simulink library "Vessel"  (R2023a)
settings: Solver=VariableStepAuto  StartTime=0.0  StopTime=10.0  RelTol=1e-3
undefined symbols (not defined in the file): A_ann_aor, alpha1, alpha2, atrium_ventricle, BSA, control, conversion_factor, DAP, DLVP, DP_close_aor, DP_open_aor, DPP, DRVP, E0, E_max, E_min, E_sa_0, E_sv_0, eta, g, K_vc_aor, K_vo_aor, l, L0, lambda, m1, m2, M_rg_aor, M_st_aor, MAP, MPP, n, P0, p_septum_on_off, p_th_on_off, phi, PVR, Q_max, rho, SAP, SI, sigma, SLVP, SPP, SRVP, SVR, t_delay, Ts, UVV_0, V0, V_0, V_max, V_tot, Y_aorta, Y_control
libraries: $bdroot x100, simulink x39, dspsigops x20, slpidlib x11, eeGeneralControl x2, dspstat3 x1
(part 1 of 4)
settings Model: Creator=emanuele  LastModifiedBy=priya
settings DataIOCC: FinalStateName=final_simstate  InitialState=new_simstate  SaveFinalState=on  SaveOperatingPoint=on
settings OptimizationCC: ReuseModelBlockBuffer=off

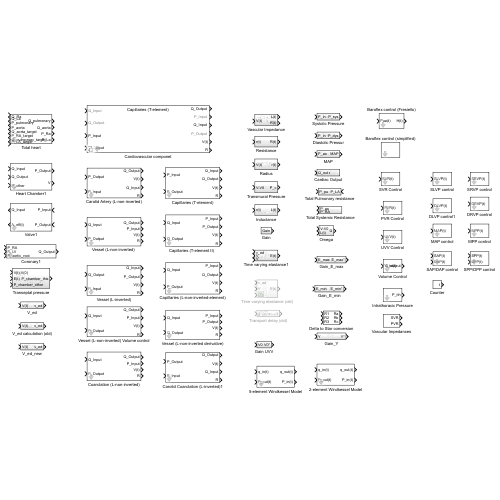
[thumbnail: Simulink's stored preview of the top-level diagram]
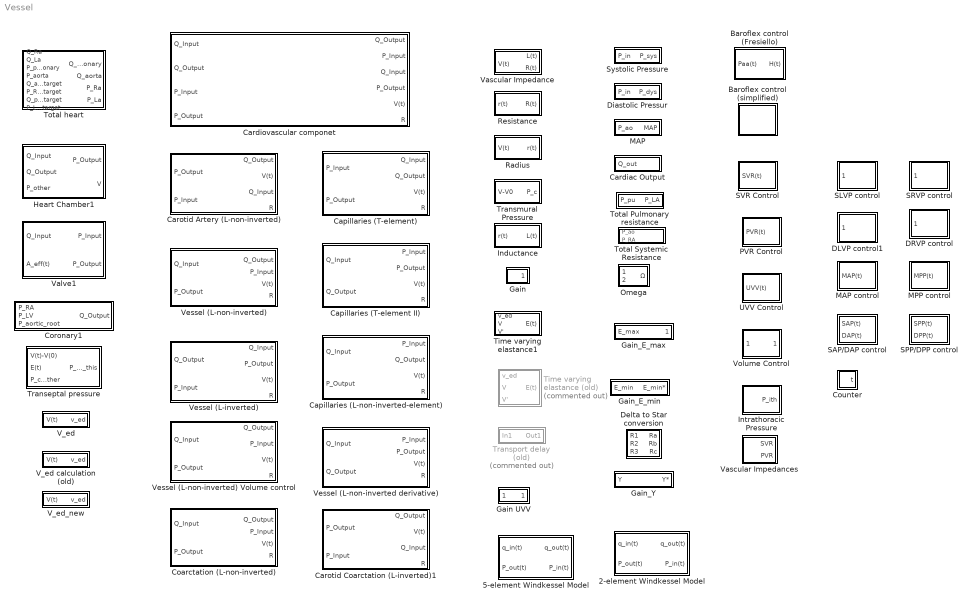
== system Vessel ==
  2-element Windkessel Model : Subsystem  mask{R1=0.001, C1=0.001}
      mask prompts: R1 "R1 (mmHg s/ml)"; C1 "C1 (ml/mmHg)"
      mask DialogControl Descr Prompt: This block models a 2-element windkessel model.
  5-element Windkessel Model : Subsystem  mask{R1=0.001, R2=0.001, C1=0.001, C2=0.001, L=0.001}
      mask prompts: R1 "R1 (mmHg s/ml)"; R2 "R2 (mmHg s/ml)"; C1 "C1 (ml/mmHg)"; C2 "C2 (ml/mmHg)"; L "L (mmHg s^2/ml)"
      mask DialogControl Descr Prompt: This block models a 5-element windkessel model.
  Baroflex control (Fresiello) : Subsystem  mask{C_Hs=-0.09, C_Hv=0.07, D_Hs=2, D_Hv=0.2, T_Hs=2, T_Hv=1.5, H_set=0.7, A=0.242, B=0.12, C=-0.041, D=-0.041, ka=11.758, kes=0.0675, kev=7.06, Fes_0=16.11, Fes_inf=2.10, Fev_0=3.2, Fev_inf0=6.3, Fas_min=2.52, Fas_max=47.78, Paa_SET0=90, tau_p=2.076, tau_z=6.37, WL=0}
      mask prompts: C_Hs "C_Hs: sympathetic control gain for the parameter H (s/(spikes/s))"; C_Hv "C_Hv: vagal control gain for the parameter H (s/(spikes/s))"; D_Hs "D_Hs: sympathetic delay for the parameter H (s)"; D_Hv "D_Hv: vagal delay for the parameter H (s)"; T_Hs "T_Hs: time constant of sympathetic control (s)"; T_Hv "T_Hv: time constant of vagal control (s)"; H_set "H_SET: set point value of H"; A "A: rate pf Paa_SET increase per unit of WL (mmHg/W)"; B "B: rate pf Fes increase per unit of WL (spike/(W⋅s))"; C "C: rate pf Fev decrease per unit of WL (spike/(W·s))"; D "D: rate of Fev_inf decrease per unit of WL (spike/(W·s))"; ka "ka: Fas slope parameter (mmHg)"; kes "kes: Fes slope parameter (s)"; kev "kev: Fev slope parameter (spikes/s)"; Fes_0 "Fes_0: Fes upper limit (spikes/s)"; Fes_inf "Fes_inf: Fes lower limit (spikes/s)"; Fev_0 "Fev_0: Fev lower limit (spikes/s)"; Fev_inf0 "Fev_inf0: Fev upper limit (spikes/s)"; Fas_min "Fas_min: lower saturation of frequency discharge (spikes/s)"; Fas_max "Fas_max: upper saturation of frequency discharge (spikes/s)"; Paa_SET0 "Paa_SET0: set point pressure (mmHg)"; tau_p "tau_p: pole (s)"; tau_z "tau_z: zero (s)"; WL "WL: workload (W)"
      mask init:
      | Fas_0 = Fas_min+Fas_max; %central point of afferent sympathetic activity (spikes/s)
      mask DialogControl DescGroupVar Prompt: Baroflex control with nerve activation function
      mask DialogControl DescTextVar Prompt: The baroreflex model was taken from Ursino (1998) and Fresiello et al. (2013). It provides a representation of the afferent nerve activity, depending on the pressure sensed in the aortic region. In addition, the model reproduces the vagal and sympathetic nerve activity and their effects on cardiovascular parameters. In the model of Ursino (1998) the pressure in the carotid arteries is the input the baroreflex control. Since in the present simulator there is no specific representation of the carotid arteries, the aortic pressure without the effect of the intrathoracic pressure was considered as input pressure for the baroreflex control (Paa).
      mask DialogControl Container5 Prompt: Baroflex parametere for cardiovasculat parameter H(t)
      mask DialogControl Container6 Prompt: General baroflex and nerve parameters
  Baroflex control (simplified) : Subsystem  mask{G_baro=0.003, P_target=110, T_target=0.7, onoff=off}
      mask prompts: G_baro "Baroflex Gain (ms/mmHg)"; P_target "Pressure target (mmHg)"; T_target "Cardiac cycle target (s)"; onoff "Enable"
      mask DialogControl noll Prompt: Baroflex Control Parameters
  Capillaries (L-non-inverted-element) : Subsystem  mask{l=0.02, r=0.0005, h=0.00001, n=11200000000, P0=6}
      mask prompts: l "Length (cm)"; r "Radius (cm)"; h "Thickness (cm)"; n "Number of branches"; P0 "P0 (mmHg)"
      mask init:
      | % rho = 1.060; % g/mL
      | % Y = 3000; % mmHg
      | % eta = 0.00024; % mmHg * s
      | % g = 980.665; % cm / s^2
      | % conversion_factor = 1.3595101283313; %g/cm^2-->mmHg
      | % lambda = 0.5;
      | % V0 = pi*r^2*l*n;
      | % E0 = Y*h/(2*pi*r^3*l*n);
      | % phi = P0/E0;
      | % R0 = eta*8*l/(pi*r^4*n);
      | % L0 = rho * l/ (pi * r^2 * n)/g/conversion_factor;
      mask DialogControl DescGroupVar Prompt: Cardiovascular vessel
      mask DialogControl DescTextVar Prompt: This block models a cardiovascular vessel. Plese choose between L-inverted elelement and not-inverted L-element. Add geomtrical information. Select what variables are input and what are outputs.
      mask DialogControl ParameterGroupVar Prompt: Vessel's Parameters
  "Capillaries (T-element II)  " : Subsystem  mask{l=0.02, r=0.0005, h=0.00001, n=11200000000, P0=6}
      mask prompts: l "Length (cm)"; r "Radius (cm)"; h "Thickness (cm)"; n "Number of branches"; P0 "P0 (mmHg)"
      mask init: same as Vessel/Capillaries (L-non-inverted-element)
      mask DialogControl DescGroupVar Prompt: Cardiovascular vessel
      mask DialogControl DescTextVar Prompt: This block models a cardiovascular vessel. Plese choose between L-inverted elelement and not-inverted L-element. Add geomtrical information. Select what variables are input and what are outputs.
      mask DialogControl ParameterGroupVar Prompt: Vessel's Parameters
  Capillaries (T-element) : Subsystem  mask{l=0.02, r=0.0005, h=0.00001, n=11200000000, P0=6}
      mask prompts: l "Length (cm)"; r "Radius (cm)"; h "Thickness (cm)"; n "Number of branches"; P0 "P0 (mmHg)"
      mask init: same as Vessel/Capillaries (L-non-inverted-element)
      mask DialogControl DescGroupVar Prompt: Cardiovascular vessel
      mask DialogControl DescTextVar Prompt: This block models a cardiovascular vessel. Plese choose between L-inverted elelement and not-inverted L-element. Add geomtrical information. Select what variables are input and what are outputs.
      mask DialogControl ParameterGroupVar Prompt: Vessel's Parameters
  Cardiac Output : Subsystem
  Cardiovascular componet : Subsystem  Variant=on  mask{choice=Capillary compartment (T element), control=None, Y_control=Systemic Arteries, l=2, r=1.6, h=0.163, n=1, P0=80, Y=2000, SI=0, V_tot=V_tot, p_th_on_off=off}
      mask prompts: choice "Windkessel model"; control "Type of control"; Y_control "Young modulus control"; l "Length (cm)"; r "Radius (cm)"; h "Thickness (cm)"; n "Number of branches"; P0 "P0 (mmHg)"; Y "Y (mmHg)"; SI "Stenosis index"; V_tot "V_tot (ml)"; p_th_on_off "Intrathoracic pressure"
      mask init:
      | rho = 1.060; % g/mL
      | %Y =2000; % mmHg
      | eta = 0.00024; % mmHg * s
      | g = 980.665; % cm / s^2
      | conversion_factor = 1.3595101283313; %g/cm^2-->mmHg
      | lambda = 0.5;
      | 
      | %  Scaling to patient's size
      | if V_tot ~=0
      |     k = r/l;                % ratio between radius and length;
      |     V_tot_0 = 4528;
      |     C = V_tot/V_tot_0;
      |     V0 = pi*r^2*l*n;        % Initial volume of original vessel
      |     l = (C*V0/pi/k^2/n)^(1/3);
      |     r = k * l;
      | end
      | 
      | % Calculate volume and impedance
      | V0 = pi*r^2*l*n;
      | E0 = 2*Y*h/(3*pi*r^3*l*n);
      | phi = P0/E0;
      | R0 = eta*8*l/(pi*r^4*n);
      | L0 = rho * l/ (pi * r^2 * n)/g/conversion_factor;
      mask TypeOptions choice: Vessel compartment (L-non-inverted element) | Vessel compartment (L-inverted element) | Capillary compartment (T element) | Capillary compartment (L-non-inverted element) | Capillary compartment (T element II) | Carotid Artery (L-non-inverted) | Vessel (L-non-inverted derivative) | Vessel (volume control)
      mask TypeOptions control: SVR control | PVR control | UVV control | None
      mask TypeOptions Y_control: Systemic Arteries | Systemic Veins | Pulmonary Arteries | Pulmonary Veins | None
      mask DialogControl DescGroupVar Prompt: Cardiovascular vessel
      mask DialogControl DescTextVar Prompt: This block models a cardiovascular vessel. Plese choose between L-inverted elelement and not-inverted L-element. Add geomtrical information. Select what variables are input and what are outputs.
      mask DialogControl ParameterGroupVar Prompt: Vessel's Parameters
  Carotid Artery (L-non-inverted) : Subsystem  mask{l=2, r=1.6, h=0.163, n=1, P0=80}
      mask prompts: l "Length (cm)"; r "Radius (cm)"; h "Thickness (cm)"; n "Number of branches"; P0 "P0 (mmHg)"
      mask init:
      | % rho = 1.060; % g/mL
      | % Y = 2000; % mmHg
      | % eta = 0.00024; % mmHg * s
      | % g = 980.665; % cm / s^2
      | % conversion_factor = 1.3595101283313; %g/cm^2-->mmHg
      | % lambda = 0.5;
      | % V0 = pi*r^2*l*n;
      | % E0 = Y*h/(2*pi*r^3*l*n);
      | % phi = P0/E0;
      | % R0 = eta*8*l/(pi*r^4*n);
      | % L0 = rho * l/ (pi * r^2 * n)/g/conversion_factor;
      mask DialogControl DescGroupVar Prompt: Cardiovascular vessel
      mask DialogControl DescTextVar Prompt: This block models a cardiovascular vessel. Plese choose between L-inverted elelement and not-inverted L-element. Add geomtrical information. Select what variables are input and what are outputs.
      mask DialogControl ParameterGroupVar Prompt: Vessel's Parameters
  Carotid Coarctation (L-inverted)1 : Subsystem  mask{l=2, SI=0, L0=0.5107007067709949, P0=100, Y=2000, Y_control=Systemic arteries}
      mask prompts: l "Length (cm)"; SI "Stenosis index"; L0 "L0 (CGS units)"; P0 "P0 (mmHg)"; Y "Young Modulus (mmhg)"; Y_control "Young modulus control"
      mask init:
      | rho = 1.060; % g/mL
      | control = 4;
      | %Y = 2000; % mmHg
      | eta = 0.00024; % mmHg * s
      | g = 980.665; % cm / s^2
      | conversion_factor = 1.3595101283313; %g/cm^2-->mmHg
      | lambda = 0.5;
      | r = sqrt(rho * l / pi / L0);
      | h = r/10;
      | n = 1;
      | V0 = pi*r^2*l;
      | E0 = Y*h/(2*pi*r^3*l);
      | phi = P0/E0;
      | R0 = eta*8*l/(pi*r^4);
      | L0 = rho * l/ (pi * r^2 )/g/conversion_factor;
      mask TypeOptions Y_control: Systemic arteries | Systemic veins | Pulmonary arteries | Pulmonary veins | None
      mask DialogControl DescGroupVar Prompt: Cardiovascular vessel
      mask DialogControl DescTextVar Prompt: This block models a cardiovascular vessel. Plese choose between L-inverted elelement and not-inverted L-element. Add geomtrical information. Select what variables are input and what are outputs.
      mask DialogControl ParameterGroupVar Prompt: Vessel's Parameters
  Coarctation (L-non-inverted) : Subsystem  mask{l=2, SI=0, L0=0.5107007067709949, P0=100, Y=Y_aorta, Y_control=Systemic Arteries}
      mask prompts: l "Length (cm)"; SI "Stenosis index"; L0 "L0 (CGS units)"; P0 "P0 (mmHg)"; Y "Young Modulus (mmhg)"; Y_control "Young Modulus control"
      mask init:
      | rho = 1.060; % g/mL
      | control = 4;
      | %Y = 2000; % mmHg
      | eta = 0.00024; % mmHg * s
      | g = 980.665; % cm / s^2
      | conversion_factor = 1.3595101283313; %g/cm^2-->mmHg
      | lambda = 0.5;
      | r = sqrt(rho * l / pi / L0);
      | h = r/10;
      | n = 1;
      | V0 = pi*r^2*l;
      | E0 = 2*Y*h/(3*pi*r^3*l);
      | phi = P0/E0;
      | R0 = eta*8*l/(pi*r^4);
      | L0 = rho * l/ (pi * r^2 )/g/conversion_factor;
      mask TypeOptions Y_control: Systemic Arteries | Systemic Veins | Pulmonary Arteries | Pulmonary Veins | None
      mask DialogControl DescGroupVar Prompt: Cardiovascular vessel
      mask DialogControl DescTextVar Prompt: This block models a cardiovascular vessel. Plese choose between L-inverted elelement and not-inverted L-element. Add geomtrical information. Select what variables are input and what are outputs.
      mask DialogControl ParameterGroupVar Prompt: Vessel's Parameters
  Coronary1 : Subsystem  mask{R_ca=0}
  Counter : Subsystem
  DLVP control1 : Subsystem  mask{DLVP_0=DLVP, dt=3, onoff=on}
      mask prompts: DLVP_0 "DLVP tartget"; dt "Time step (s)"; onoff "Enable"
  DRVP control : Subsystem  mask{DRVP_0=DRVP, dt=3, onoff=on}
      mask prompts: DRVP_0 "DRVP tartget"; dt "Time step (s)"; onoff "Enable"
  Delta to Star conversion : Subsystem
  Diastolic Pressur : Subsystem
  Gain : Subsystem
  Gain UVV : Subsystem
  Gain_E_max : Subsystem
  Gain_E_min : Subsystem
  Gain_Y : Subsystem
  Heart Chamber1 : Subsystem  mask{control=Right Atrium, E_max=0.06, E_min=0.04, alpha1=0.1, alpha2=0.2, m1=1.2, m2=10, R_wall=0.0005, t_delay=85e-3, V_0=17, v_o=40, sigma=0.0015, V_max=400, Q_max=2000, T0=0.8, P_pc_0=-2, K_pc=1, V_pc_0=320, V_pe=30, phi_pc=40, E_sa_0=12, E_sv_0=46, atrium_ventricle=Atrium}
      mask prompts: E_max "Maximum elastance (mmHg/mL)"; E_min "Minimum elastance (mmHg/mL)"; alpha1 "α₁"; alpha2 "α₂"; m1 "m₁"; m2 "m₂"; V_0 "Residual volume (mL)"; v_o "Initial volume (mL)"; sigma "σ"; T0 "Cardiac cycle (s)"; P_pc_0 "P_pc₀ (minimal pericardial pressure)"; K_pc "K_pc (pericardial pressure constant"; V_pc_0 "V_pc (pericardial volume constant)"; V_pe "Pericardial fluid volume"; phi_pc "φ_pc (pericardial volume constant)"; E_sa_0 "E_sa₀"; E_sv_0 "E_sv₀"; atrium_ventricle "Chamber"
      mask init:
      | %tau1 = alpha1*T0;
      | %tau2 = alpha2*T0;
      | Q_min = -Q_max;
      | V_min = V_0;
      mask TypeOptions control: Right Atrium | Right Ventricle | Left Atrium | Left Ventricle | None
      mask TypeOptions atrium_ventricle: Atrium | Ventricle
      mask DialogControl ParameterGroupVar Prompt: Heart Chamber Parameters
      mask DialogControl Container4 Prompt: Pericardium Parameters
  Inductance : Subsystem
  Intrathoracic Pressure : Subsystem  mask{t_ins=2, t_exp=3, p_ita=1.8, p_itb=-5.5}
      mask prompts: t_ins "Inspiration cycle (s)"; t_exp "Expiration cycle (s)"; p_ita "Pressure variation (mmHg)"; p_itb "Pressure baseline (mmHg)"
      mask init:
      | tau_insp = t_ins/10;
      | tau_exp = t_exp/10;
      mask DialogControl DescGroupVar Prompt: Intrathoracic pressure
      mask DialogControl DescTextVar Prompt: The parameters for simulating the varying thoracic pressure during the breathing cycle are taken from: A comprehensive model for right-left heart interaction under the influence of pericardium and baroreflex
  MAP : Subsystem
  MAP control : Subsystem  mask{MAP_0=MAP, dt=1, onoff=on}
      mask prompts: MAP_0 "MAP tartget"; dt "Time step (s)"; onoff "Enable"
  MPP control : Subsystem  mask{MPP_0=MPP, dt=3, onoff=on}
      mask prompts: MPP_0 "MPP tartget"; dt "Time step (s)"; onoff "Enable"
  Omega : Subsystem
  PVR Control : Subsystem  mask{PVR_0=PVR, onoff=on}
      mask prompts: PVR_0 "PVR tartget"; onoff "Enable"
  Radius : Subsystem
  Resistance : Subsystem
  SAP/DAP control : Subsystem  mask{SAP_0=SAP, DAP_0=DAP, dt=1, onoff=on}
      mask prompts: SAP_0 "SAP target"; DAP_0 "DAP target"; dt "Time step (s)"; onoff "Enable"
  SLVP control : Subsystem  mask{SLVP_0=SLVP, dt=3, onoff=on}
      mask prompts: SLVP_0 "SLVP tartget"; dt "Time step (s)"; onoff "Enable"
  SPP/DPP control : Subsystem  mask{SPP_0=SPP, DPP_0=DPP, dt=3, onoff=on}
      mask prompts: SPP_0 "SPP target"; DPP_0 "DPP target"; dt "Time step (s)"; onoff "Enable"
  SRVP control : Subsystem  mask{SRVP_0=SRVP, dt=3, onoff=on}
      mask prompts: SRVP_0 "SRVP tartget"; dt "Time step (s)"; onoff "Enable"
  SVR Control : Subsystem  mask{SVR_0=SVR, onoff=on}
      mask prompts: SVR_0 "SVR tartget"; onoff "Enable"
  Systolic Pressure : Subsystem
  Time varying elastance (old) : Subsystem  Commented=on
  Time varying elastance1 : Subsystem
  Total Pulmonary resistance : Subsystem
      settings: PortSchema="{\"entries\":[{\"content\":{\"sides\":[{\"content\":{\"connectorIds\":[\"In1\"]},\"type\":\"ConnectorPlacement.EquallySpacedRectSide\",\"uuid\":\"c9341461-c171-4eac-a287-36e7cd79ba9c\"},{\"content\":{\"connectorIds\":[\"In2\"],\"side\":\"RIGHT\"},\"type\":\"ConnectorPlacement.EquallySpacedRectSide\",\"uuid\":\"dd479575-dfa7-40be-8840-552306c7a812\"},{\"content\":{\"connectorIds\":[],\"side\":\"TOP\"},\"type\":\"ConnectorPlacement.EquallySpacedRectSide\",\"uuid\":\"55fb924b-6719-416a-80e5-0f49fb901268\"}]},\"type\":\"ConnectorPlacement.EquallySpacedConnector\",\"uuid\":\"ed4dd8c3-ddc7-4a34-b37b-80f1af9032bf\"}],\"packageUris\":[\"http://schema.mathworks.com/mf0/Connector/R2020b\"],\"version\":\"1.0\"}"
  Total Systemic Resistance : Subsystem
  Total heart : Subsystem  mask{BSA=BSA, T0=0.833, R_lca=40, R_rca=80, p_septum_on_off=on, E_max_ra=0.15, E_max_rv=0.6, E_max_la=0.17, E_max_lv=3, E_min_ra=0.04, E_min_rv=0.04, E_min_la=0.08, E_min_lv=0.09, alpha1_ra=0.1, alpha1_rv=0.2, alpha1_la=0.1, alpha1_lv=0.2, alpha2_ra=0.2, alpha2_rv=0.25, alpha2_la=0.2, alpha2_lv=0.25, m1_ra=1.2, m1_rv=1.2, m1_la=1.2, m1_lv=1.2, m2_ra=10, m2_rv=10, m2_la=10, m2_lv=20, R_wall_ra=0.0005, R_wall_rv=0.00020, R_wall_la=0.00050, R_wall_lv=0.00005, t_delay_ra=85e-3, t_delay_rv=245e-3, t_delay_la=95e-3, t_delay_lv=245e-3, V_0_ra=17, V_0_rv=55, V_0_la=3, V_0_lv=5, v_o_ra=60, v_o_rv=100, v_o_la=60, v_o_lv=40, sigma_ra=0.0015, sigma_rv=0.0030, sigma_la=0.0015, sigma_lv=0.003, V_max_ra=400, V_max_rv=400, V_max_la=400, V_max_lv=400, Q_max_ra=4000, Q_max_rv=2000, Q_max_la=4000, Q_max_lv=2000, A_ann_tri=7.7, A_ann_pul=1.5^2*pi, A_ann_mit=7.7, A_ann_aor=1.6^2*pi, K_vo_tri=40, K_vo_pul=30, K_vo_mit=40, K_vo_aor=20, K_vc_tri=30, K_vc_pul=30, K_vc_mit=20, K_vc_aor=20, M_st_tri=1, M_st_pul=1, M_st_mit=1, M_st_aor=1, M_rg_tri=0, M_rg_pul=0, M_rg_mit=0, M_rg_aor=0, DP_open_tri=0, DP_open_pul=0, DP_open_mit=0, DP_open_aor=0, DP_close_tri=0, DP_close_pul=0, DP_close_mit=0, DP_close_aor=0, P_pc_0=-2, K_pc=1, V_pc_0=320, V_pe=30, phi_pc=50, E_sa_0=12, E_sv_0=46}
      mask prompts: BSA "BSA (m^2)"; T0 "Cardiac cycle (s)"; R_lca "Left coronary artery resistance"; R_rca "Right coronary artery resistance"; p_septum_on_off "Atrial/Ventricular septum"; P_pc_0 "P_pc₀ (minimal pericardial pressure)"; K_pc "K_pc (pericardial pressure constant"; V_pc_0 "V_pc (pericardial volume constant)"; V_pe "Pericardial fluid volume"; phi_pc "φ_pc (pericardial volume constant)"; E_sa_0 "E_sa₀"; E_sv_0 "E_sv₀"
      mask init:
      | %General
      | if BSA~=0
      |     
      | V_0_ra      =   BSA^(1.0974) * 5.1668;
      | V_0_rv      =   BSA^(1.0974) * 5.1668;
      | 
      | sigma_ra    =   BSA^(-1.0849) * 0.0029;
      | sigma_la    =   BSA^(-1.0849) * 0.0029;
      | sigma_rv    =   BSA^(-1.0522) * 0.0188;
      | sigma_lv    =   BSA^(-1.0522) * 0.0188;
      | 
      | V_max_ra    =   BSA^(1.0971) * 129.3569;
      | V_max_la    =   BSA^(1.0971) * 129.3569;
      | V_max_rv    =   BSA^(1.0956) * 181.1664;
      | V_max_lv    =   BSA^(1.0956) * 181.1664;
      | 
      | Q_max_ra    =   BSA^(1.0955) * 2070.9;
      | Q_max_la    =   BSA^(1.0955) * 2070.9;
      | Q_max_rv    =   BSA^(1.0965) * 1034.8;
      | Q_max_lv    =   BSA^(1.0965) * 1034.8;
      | 
      | V_pe        =   BSA^(1.1720) * 14.7750;
      | V_pc_0      =   BSA^(1.3765) * 127.1945;
      | phi_pc      =   BSA^(1.1152) * 25.6292;
      | E_sa_0      =   BSA^(-1.0014) * 18.5433;
      | E_sv_0      =   BSA^(-1.0014) * 18.5433;
      | 
      | end
      mask DialogControl Container7 Prompt: General Parameters
      mask DialogControl Container9 Prompt: General Parameters
      mask DialogControl Container8 Prompt: Chambers parameters
      mask DialogControl Container15 Prompt: Chambers parameters
      mask DialogControl Control1_copy_copy_copy_copy_copy_copy Prompt: Parameter
      mask DialogControl Control1_copy_copy_copy Prompt: Right atrium
      mask DialogControl Control1_copy_copy_copy_copy Prompt: Right ventricle
      mask DialogControl Control1_copy_copy_copy_copy_copy Prompt: Left Atrium
      mask DialogControl Control1_copy Prompt: Left Ventricle
      mask DialogControl Control6 Prompt: E_max
      mask DialogControl Control7 Prompt: E_min
      mask DialogControl Control8 Prompt: α₁
      mask DialogControl Control9 Prompt: α₂
      mask DialogControl Control10 Prompt: m₁
      mask DialogControl Control11 Prompt: m₂
      mask DialogControl Control12 Prompt: R_wall
      mask DialogControl Control13 Prompt: t_delay
      mask DialogControl Control14 Prompt: V₀
      mask DialogControl Control15 Prompt: v₀
      mask DialogControl Control16 Prompt: σ
      mask DialogControl Control15_copy Prompt: V_max
      mask DialogControl Control15_copy_copy Prompt: Q_max
      mask DialogControl Container10 Prompt: Valves Parameters
      mask DialogControl Container5 Prompt: Valves Parameters
      mask DialogControl Control17 Prompt: Parameter
      mask DialogControl Control18 Prompt: Tricuspid valve
      mask DialogControl Control18_copy Prompt: Pulmonary valve
      mask DialogControl Control18_copy_copy Prompt: Mitral valve
      mask DialogControl Control18_copy_copy_copy Prompt: Aortic valve
      mask DialogControl Control22 Prompt: A_ann
      mask DialogControl Control23 Prompt: K_vo
      mask DialogControl Control24 Prompt: K_vc
      mask DialogControl Control25 Prompt: M_st
      mask DialogControl Control26 Prompt: M_rg
      mask DialogControl Control27 Prompt: Δp_open
      mask DialogControl Control28 Prompt: Δp_close
      mask DialogControl Container11 Prompt: Pericardium Parameters
      mask DialogControl Container4 Prompt: Pericardium Parameters
  Transeptal pressure : Subsystem
  Transmural Pressure : Subsystem
  Transport delay (old) : Subsystem  Commented=on
  UVV Control : Subsystem  mask{UVV_0=3400, onoff=on}
      mask prompts: UVV_0 "UVV tartget"; onoff "Enable"
  V_ed : Subsystem
  V_ed calculation (old) : Subsystem
  V_ed_new : Subsystem
  Valve1 : Subsystem  mask{A_ann=A_ann_aor, K_vo=K_vo_aor, K_vc=K_vc_aor, M_st=M_st_aor, M_rg=M_rg_aor, DP_open=DP_open_aor, DP_close=DP_close_aor, Q_max=4000, Q_min=0}
      mask prompts: A_ann "Area (cm^2)"; K_vo "Opening constant (1/mmHg/s)"; K_vc "Closing constant (1/mmHg/s)"; M_st "Stenosis index"; M_rg "Regurgitation index"; DP_open "Opening pressure gradient (mmHg)"; DP_close "Closing pressure gradient (mmHg)"; Q_max "Maximum flow"; Q_min "Minimum flow"
      mask init:
      | rho = 1.060; %g/cm^3
  Vascular Impedance : Subsystem
  Vascular Impedances : Subsystem
  Vessel (L-inverted) : Subsystem  mask{l=2, r=1.6, h=0.163, n=1, P0=80}
      mask prompts: l "Length (cm)"; r "Radius (cm)"; h "Thickness (cm)"; n "Number of branches"; P0 "P0 (mmHg)"
      mask init: same as Vessel/Capillaries (L-non-inverted-element)
      mask DialogControl DescGroupVar Prompt: Cardiovascular vessel
      mask DialogControl DescTextVar Prompt: This block models a cardiovascular vessel. Plese choose between L-inverted elelement and not-inverted L-element. Add geomtrical information. Select what variables are input and what are outputs.
      mask DialogControl ParameterGroupVar Prompt: Vessel's Parameters
  Vessel (L-non-inverted derivative) : Subsystem  mask{l=2, r=1.6, h=0.163, n=1, P0=80}
      mask prompts: l "Length (cm)"; r "Radius (cm)"; h "Thickness (cm)"; n "Number of branches"; P0 "P0 (mmHg)"
      mask init:
      | % rho = 1.060; % g/mL
      | % Y = 3000; % mmHg
      | % eta = 0.00024; % mmHg * s
      | % g = 980.665; % cm / s^2
      | % conversion_factor = 1.3595101283313; %g/cm^2-->mmHg
      | % lambda = 0.5;
      | % V0 = pi*r^2*l*n;
      | % E0 = Y*h/(2*pi*r^3*l*n);
      | % phi = P0/E0;
      | % R0 = eta*8*l/(pi*r^4*n);
      | % L0 = rho * l/ (pi * r^2 * n)/g/conversion_factor;
      mask DialogControl DescGroupVar Prompt: Cardiovascular vessel
      mask DialogControl DescTextVar Prompt: This block models a cardiovascular vessel. Plese choose between L-inverted elelement and not-inverted L-element. Add geomtrical information. Select what variables are input and what are outputs.
      mask DialogControl ParameterGroupVar Prompt: Vessel's Parameters
  "Vessel (L-non-inverted) " : Subsystem  mask{l=2, r=1.6, h=0.163, n=1, P0=80}
      mask prompts: l "Length (cm)"; r "Radius (cm)"; h "Thickness (cm)"; n "Number of branches"; P0 "P0 (mmHg)"
      mask init: same as Vessel/Vessel (L-non-inverted derivative)
      mask DialogControl DescGroupVar Prompt: Cardiovascular vessel
      mask DialogControl DescTextVar Prompt: This block models a cardiovascular vessel. Plese choose between L-inverted elelement and not-inverted L-element. Add geomtrical information. Select what variables are input and what are outputs.
      mask DialogControl ParameterGroupVar Prompt: Vessel's Parameters
  Vessel (L-non-inverted) Volume control : Subsystem  mask{l=2, r=1.6, h=0.163, n=1, P0=80}
      mask prompts: l "Length (cm)"; r "Radius (cm)"; h "Thickness (cm)"; n "Number of branches"; P0 "P0 (mmHg)"
      mask init: same as Vessel/Vessel (L-non-inverted derivative)
      mask DialogControl DescGroupVar Prompt: Cardiovascular vessel
      mask DialogControl DescTextVar Prompt: This block models a cardiovascular vessel. Plese choose between L-inverted elelement and not-inverted L-element. Add geomtrical information. Select what variables are input and what are outputs.
      mask DialogControl ParameterGroupVar Prompt: Vessel's Parameters
  Volume Control : Subsystem  mask{V_tot_0=4800}
      mask prompts: V_tot_0 "Total blood volume (mL)"

== system Vessel/2-element Windkessel Model ==
  note: 2-element Windkessel Model
  q_in(t) : Inport
  P_out(t) : Inport  Port=2
  Bias : Bias  Bias=0.0  SaturateOnIntegerOverflow=off
  Gain3 : Gain  Gain=1/C1
  Gain4 : Gain  Gain=1/R1
  Minus3 : Sum  Inputs=+-
  Minus4 : Sum  Inputs=-+
  P_1(t) : Integrator
  q_out(t) : Outport
  P_in(t) : Outport  Port=2
  wires:
  Minus4/1 -> Gain4/1
  P_out(t)/1 -> Minus4/1  "P_out(t)"
  P_1(t)/1 -> Bias/1  "P_1(t)"
  Gain3/1 -> P_1(t)/1  "P_1(t)'"
  Minus3/1 -> Gain3/1  "q_1(t)"
  Gain4/1 -> Minus3/2, q_out(t)/1  "q_out(t)"
  q_in(t)/1 -> Minus3/1  "q_in(t)"
  Bias/1 -> P_in(t)/1, Minus4/2

== system Vessel/5-element Windkessel Model ==
  note: 5-element Windkessel Model
  q_in(t) : Inport
  P_out(t) : Inport  Port=2
  Bias : Bias  Bias=0.0  SaturateOnIntegerOverflow=off
  Bias1 : Bias  Bias=0.0  SaturateOnIntegerOverflow=off
  Gain : Gain  Gain=R1
  Gain1 : Gain  Gain=1/C1
  Gain2 : Gain  Gain=1/L
  Gain3 : Gain  Gain=1/C2
  Gain4 : Gain  Gain=1/R2
  Minus : Sum  Inputs=-+
  Minus1 : Sum
  Minus2 : Sum  Inputs=+-
  Minus3 : Sum  Inputs=+-
  Minus4 : Sum  Inputs=-+
  P_2(t) : Integrator
  P_C1(t) : Integrator
  Unit Delay : UnitDelay  SampleTime=-1  HasFrameUpgradeWarning=on
  q_L(t) : Integrator
  q_out(t) : Outport
  P_in(t) : Outport  Port=2
  wires:
  Minus/1 -> Gain1/1, Gain/1  "q_1(t)"
  q_in(t)/1 -> Minus/2  "q_in(t)"
  P_C1(t)/1 -> Bias1/1  "P_C1(t)"
  Gain/1 -> Unit Delay/1  "P_R1(t)"
  Gain1/1 -> P_C1(t)/1  "P_C1(t)'"
  Minus1/1 -> P_in(t)/1, Minus2/1  "P_1(t)"
  Minus2/1 -> Gain2/1  "P_1(t)"
  Gain2/1 -> q_L(t)/1  "q_L(t)'"
  q_L(t)/1 -> Minus3/1, Minus/1  "q_L(t)"
  Gain4/1 -> q_out(t)/1, Minus3/2  "q_out(t)"
  Minus3/1 -> Gain3/1  "q_2(t)"
  Gain3/1 -> P_2(t)/1  "P_2(t)'"
  P_2(t)/1 -> Bias/1  "P_2(t)"
  P_out(t)/1 -> Minus4/1  "P_out(t)"
  Minus4/1 -> Gain4/1  "q_out(t)"
  Unit Delay/1 -> Minus1/2
  Bias/1 -> Minus4/2, Minus2/2
  Bias1/1 -> Minus1/1

== system Vessel/Baroflex control (Fresiello) ==
  Paa(t) : Inport
  Afferent sympathetic activity : Subsystem
  Constant : Constant  Value=H_set
  Efferent sympathetic nerve activity : Subsystem
  Efferent vagal nerve activity : Subsystem
  Gain : Gain  Gain=1/T_Hs
  Gain1 : Gain  Gain=1/T_Hv
  Integrator : Integrator
  Integrator1 : Integrator
  Minus : Sum  Inputs=-+|
  Minus1 : Sum  Inputs=+++
  Minus2 : Sum  Inputs=|+-
  Pressure derivation : Subsystem
  Static sympathetic function : Subsystem
  Static vagal function : Subsystem
  XY Graph : Record  FileSettingsInternal="{\"entries\":[{\"content\":{\"excelSettings\":{\"content\":{},\"type\":\"Streamout.ExcelSettings\"}},\"type\":\"Streamout.FileSettingStorage\",\"uuid\":\"\"}],\"packageUris\":[\"http:\\/\\/schema.mathworks.com\\/mf0\\/streamout_blocks\\/R2020a\"],\"version\":\"1.0\"}"  Layout=[1 1]  SignalsInternal="{\"entries\":[{\"content\":{\"signals\":[{\"content\":{\"blockPath\":[],\"dimensions\":[1],\"domain\":\"\",\"lineColor\":\"#a2142f\",\"plots\":[1],\"port\":1,\"signalID\":8,\"signalName\":\"XY Graph:1\"},\"type\":\"RecordBlkView.Signal\",\"uuid\":\"\"},{\"content\":{\"blockPath\":[],\"dimensions\":[1],\"domain\":\"\",\"lineColor\":\"#139fff\",\"plots\":[1],\"port\":2,\"signalID\":11,\"signalName\":\"XY Graph:2\"},\"type\":\"RecordBlkView.Signal\",\"uuid\":\"\"}]},\"type\":\"RecordBlkView.InputSignals\",\"uuid\":\"\"}],\"packageUris\":[\"http:\\/\\/schema.mathworks.com\\/mf0\\/streamout_blocks\\/R2020a\"],\"version\":\"1.0\"}"  VisualizationBindings="{\"xyplotplugin\":{\"info\":[{\"series\":[{\"bindingParametersList\":[{\"parameter\":\"X-Axis\",\"signalID\":8,\"signalName\":\"XY Graph:1\"},{\"parameter\":\"Y-Axis\",\"signalID\":11,\"signalName\":\"XY Graph:2\"}],\"seriesID\":30739}],\"subplotID\":1}]}}"  CompatibilityTag=XY
  H(t) : Outport
  wires:
  Minus1/1 -> H(t)/1
  Constant/1 -> Minus1/2
  Minus/1 -> Gain/1
  Integrator/1 -> Minus/1, Minus1/1  "ΔH_s(t)"
  Static sympathetic function/1(sf_Hs(t)) -> Minus/2  "sf_Hs(t)"
  Gain/1 -> Integrator/1  "ΔH_s(t)'"
  Gain1/1 -> Integrator1/1  "ΔH_v(t)'"
  Static vagal function/1(sf_Hv(t)) -> Minus2/1  "sf_Hv(t)"
  Integrator1/1 -> Minus1/3, Minus2/2  "ΔH_v(t)"
  Minus2/1 -> Gain1/1
  Efferent sympathetic nerve activity/1(" Fes(t)") -> Static sympathetic function/1(Fes(t))  "Fes(t)"
  Efferent vagal nerve activity/1(" Fev(t)") -> Static vagal function/1(Fev(t))  "Fev(t)"
  Afferent sympathetic activity/1(Fas(t)) -> XY Graph/1, Efferent sympathetic nerve activity/1(Fas(t)), Efferent vagal nerve activity/1(Fas(t))
  Pressure derivation/1(P(t)) -> XY Graph/2, Afferent sympathetic activity/1(P(t))
  Paa(t)/1 -> Pressure derivation/1(Paa(t))

== system Vessel/Baroflex control (simplified) ==
  Constant : Constant  Value=P_target
  Constant1 : Constant  Value=T_target
  Constant2 : Constant  Value=onoff
  Data Store Read : DataStoreRead  DataStoreName=T  IndexOptions=Index vector (dialog)  Indices=1  OutputSizes=1
  Data Store Write : DataStoreWrite  DataStoreName=T  IndexOptions=Index vector (dialog)  Indices=1  OutputSizes=1
  Gain : Gain  Gain=G_baro
  Minus : Sum  Inputs=+-
  Minus1 : Sum
  Switch : Switch  Criteria=u2 > Threshold  SaturateOnIntegerOverflow=off  InputSameDT=off
  wires:
  Minus1/1 -> Switch/1
  [P_sys] -> Minus/1
  Constant/1 -> Minus/2
  Gain/1 -> Minus1/1
  Constant1/1 -> Minus1/2
  Minus/1 -> Gain/1
  Constant2/1 -> Switch/2
  Data Store Read/1 -> Switch/3
  Switch/1 -> Data Store Write/1

== system Vessel/Capillaries (L-non-inverted-element) ==
  Q_Input : Inport
  P_Output : Inport  Port=2  Unit=mmHg
  "   " : Sum  Inputs=-+
  Add : Sum  Inputs=+-
  Add1 : Sum  Inputs=+++
  Constant1 : Constant  Value=V0
  Delay : Delay  DelayLength=1
  Divide : Product  Inputs=*/
  Gain UVV : $bdroot/Gain UVV  SystemSampleTime=-1  VariantActivationTime=update diagram  Latency=0  AutoFrameSizeCalculation=off
  Gain1 : Gain  Gain=p_th_on_off
  IC : InitialCondition  Value=0
  IC1 : InitialCondition  Value=P0
  IC2 : InitialCondition  Value=0
  Integrator : Integrator  InitialConditionSource=external  LimitOutput=on  LowerSaturationLimit=0  ContinuousStateAttributes='Volume'
  Omega : $bdroot/Omega  SystemSampleTime=-1  VariantActivationTime=update diagram  Latency=0  AutoFrameSizeCalculation=off
  Product4 : Product
  Saturation : Saturate  UpperLimit=4000  LowerLimit=-4000
  Subtract : Sum  Inputs=+-
  Transmural Pressure : $bdroot/Transmural Pressure  SystemSampleTime=-1  VariantActivationTime=update diagram  Latency=0  AutoFrameSizeCalculation=off
  Vascular Impedance : $bdroot/Vascular Impedance  SystemSampleTime=-1  VariantActivationTime=update diagram  Latency=0  AutoFrameSizeCalculation=off
  P_Input : Outport
  Q_Output : Outport  Port=2
  V(t) : Outport  Port=3
  R : Outport  Port=4
  wires:
  "   "/1 -> Integrator/1, IC2/1  "V(t)'"
  Integrator/1 -> V(t)/1, Add/1  "V(t)"
  Add/1 -> Transmural Pressure/1  "V-V0"
  Transmural Pressure/1 -> Add1/1  "P_c"
  Product4/1 -> Add1/2  "P_Ω"
  Omega/1 -> Product4/1  "Ω"
  Add1/1 -> IC1/1, Subtract/1
  P_Output/1 -> Subtract/2
  Subtract/1 -> Divide/1
  Constant1/1 -> Gain UVV/1
  Divide/1 -> Saturation/1, Delay/1
  [P_ith] -> Gain1/1
  Gain1/1 -> Add1/3
  IC1/1 -> P_Input/1
  IC/1 -> "   "/1
  IC2/1 -> Product4/2
  Delay/1 -> IC/1
  Saturation/1 -> Q_Output/1
  Q_Input/1 -> "   "/2
  Vascular Impedance/2 -> R/1, Divide/2
  Gain UVV/1 -> Integrator/2, Vascular Impedance/1, Add/2

== system Vessel/Capillaries (T-element II)   ==
  "Q_Input " : Inport  Unit=mL/s
  "Q_Output " : Inport  Port=2  Unit=mL/s
  "   " : Sum  Inputs=+-
  Add : Sum  Inputs=+-
  Add1 : Sum
  Add2 : Sum  Inputs=+-
  Add3 : Sum
  Constant1 : Constant  Value=V0
  Delay : Delay  DelayLength=1
  Gain UVV : $bdroot/Gain UVV  SystemSampleTime=-1  VariantActivationTime=update diagram  Latency=0  AutoFrameSizeCalculation=off
  Gain2 : Gain  Gain=1/2
  IC : InitialCondition  Value=0
  Integrator : Integrator  InitialConditionSource=external  LimitOutput=on  LowerSaturationLimit=0  ContinuousStateAttributes='Volume'
  Omega : $bdroot/Omega  SystemSampleTime=-1  VariantActivationTime=update diagram  Latency=0  AutoFrameSizeCalculation=off
  Product : Product
  Product1 : Product
  Product4 : Product
  Transmural Pressure : $bdroot/Transmural Pressure  SystemSampleTime=-1  VariantActivationTime=update diagram  Latency=0  AutoFrameSizeCalculation=off
  Vascular Impedance : $bdroot/Vascular Impedance  SystemSampleTime=-1  VariantActivationTime=update diagram  Latency=0  AutoFrameSizeCalculation=off
  P_Input : Outport
  P_Output : Outport  Port=2  Unit=mmHg
  V(t) : Outport  Port=3
  R : Outport  Port=4
  wires:
  Add2/1 -> P_Output/1
  Add3/1 -> P_Input/1
  "Q_Output "/1 -> Product/1, "   "/2
  "Q_Input "/1 -> "   "/1, Product1/1
  "   "/1 -> Integrator/1, IC/1  "V(t)'"
  Integrator/1 -> Add/1, V(t)/1  "V(t)"
  Add/1 -> Transmural Pressure/1  "V-V0"
  Add1/1 -> Add3/2, Add2/1
  Transmural Pressure/1 -> Add1/1  "P_c"
  Product4/1 -> Add1/2  "P_Ω"
  Omega/1 -> Product4/1  "Ω"
  Constant1/1 -> Gain UVV/1
  Product1/1 -> Add3/1
  Product/1 -> Add2/2
  Delay/1 -> Product4/2
  IC/1 -> Delay/1
  Gain2/1 -> Product1/2, Product/2
  Vascular Impedance/2 -> R/1, Gain2/1
  Gain UVV/1 -> Vascular Impedance/1, Add/2, Integrator/2

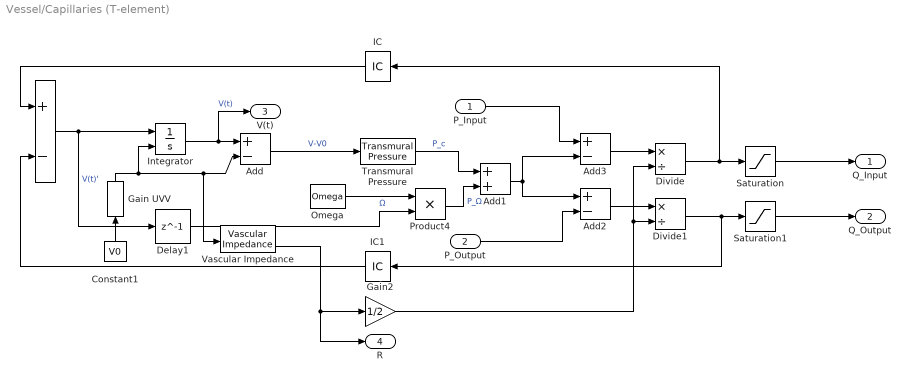
== system Vessel/Capillaries (T-element) ==
  P_Input : Inport
  P_Output : Inport  Port=2
  "   " : Sum  Inputs=+-
  Add : Sum  Inputs=+-
  Add1 : Sum
  Add2 : Sum  Inputs=+-
  Add3 : Sum  Inputs=+-
  Constant1 : Constant  Value=V0
  Delay1 : Delay  DelayLength=1
  Divide : Product  Inputs=*/
  Divide1 : Product  Inputs=*/
  Gain UVV : $bdroot/Gain UVV  SystemSampleTime=-1  VariantActivationTime=update diagram  Latency=0  AutoFrameSizeCalculation=off
  Gain2 : Gain  Gain=1/2
  IC : InitialCondition  Value=0
  IC1 : InitialCondition  Value=0
  Integrator : Integrator  InitialConditionSource=external  LimitOutput=on  LowerSaturationLimit=0  ContinuousStateAttributes='Volume'
  Omega : $bdroot/Omega  SystemSampleTime=-1  VariantActivationTime=update diagram  Latency=0  AutoFrameSizeCalculation=off
  Product4 : Product
  Saturation : Saturate  UpperLimit=4000  LowerLimit=-4000
  Saturation1 : Saturate  UpperLimit=4000  LowerLimit=-4000
  Transmural Pressure : $bdroot/Transmural Pressure  SystemSampleTime=-1  VariantActivationTime=update diagram  Latency=0  AutoFrameSizeCalculation=off
  Vascular Impedance : $bdroot/Vascular Impedance  SystemSampleTime=-1  VariantActivationTime=update diagram  Latency=0  AutoFrameSizeCalculation=off
  Q_Input : Outport
  Q_Output : Outport  Port=2  Unit=mmHg
  V(t) : Outport  Port=3
  R : Outport  Port=4
  wires:
  Constant1/1 -> Gain UVV/1
  Omega/1 -> Product4/1  "Ω"
  Product4/1 -> Add1/2  "P_Ω"
  Transmural Pressure/1 -> Add1/1  "P_c"
  Add1/1 -> Add2/1, Add3/2
  Add/1 -> Transmural Pressure/1  "V-V0"
  Integrator/1 -> V(t)/1, Add/1  "V(t)"
  "   "/1 -> Delay1/1, Integrator/1  "V(t)'"
  Add3/1 -> Divide/1
  Add2/1 -> Divide1/1
  IC/1 -> "   "/1
  IC1/1 -> "   "/2
  P_Input/1 -> Add3/1
  P_Output/1 -> Add2/2
  Delay1/1 -> Product4/2
  Gain2/1 -> Divide1/2, Divide/2
  Divide/1 -> Saturation/1, IC/1
  Divide1/1 -> Saturation1/1, IC1/1
  Saturation1/1 -> Q_Output/1
  Saturation/1 -> Q_Input/1
  Vascular Impedance/2 -> R/1, Gain2/1
  Gain UVV/1 -> Vascular Impedance/1, Add/2, Integrator/2

== system Vessel/Cardiac Output ==
  Q_out : Inport
  Data Store Read1 : DataStoreRead  DataStoreName=T  IndexOptions=Index vector (dialog)  Indices=1  OutputSizes=1
  Divide : Product  Inputs=/*
  Gain2 : Gain  Gain=60
  Integrator1 : Integrator  ExternalReset=falling
  Pulse Generator : DiscretePulseGenerator  PulseType=Time based  TimeSource=Use external signal  Period=100  PulseWidth=1e-3
  Sample and Hold : dspsigops/Sample and Hold  trig=Rising edge  initCond=0  latchinput=off
  To Workspace1 : ToWorkspace  VariableName=SV  SampleTime=-1
  To Workspace4 : ToWorkspace  VariableName=CO  SampleTime=-1
  tag scope: CO=global, Stroke_volume=global
  wires:
  Divide/1 -> [CO], To Workspace4/1
  Data Store Read1/1 -> Divide/1
  Gain2/1 -> Divide/2
  Q_out/1 -> Integrator1/1
  Pulse Generator/1 -> Sample and Hold/Trigger, Integrator1/2
  [t_b] -> Pulse Generator/1
  Integrator1/1 -> Sample and Hold/1
  Sample and Hold/1 -> [Stroke_volume], To Workspace1/1, Gain2/1

== system Vessel/Cardiovascular componet ==
  note: 1) Add Subsystem or Model blocks as valid variant choices.
      | 2) You cannot connect blocks at this level. At simulation, connectivity is automatically
      | determined, based on the active variant and port name matching.
  Q_Input : Inport
  Q_Output : Inport  Port=2
  P_Input : Inport  Port=3
  P_Output : Inport  Port=4
  Capillaries (L-non-inverted-element) : $bdroot/Capillaries (L-non-inverted-element)  VariantControl=choice == 4  l=l  r=r  h=h  n=n  P0=P0
  "Capillaries (T-element II)  " : $bdroot/Capillaries (T-element II)    VariantControl=choice == 5  l=l  r=r  h=h  n=n  P0=P0
  Capillaries (T-element) : $bdroot/Capillaries (T-element)  VariantControl=choice == 3  l=l  r=r  h=h  n=n  P0=P0
  Carotid Artery (L-non-inverted) : $bdroot/Carotid Artery (L-non-inverted)  VariantControl=choice == 6  l=l  r=r  h=h  n=n  P0=P0
  Vessel (L-inverted) : $bdroot/Vessel (L-inverted)  VariantControl=choice == 2  l=l  r=r  h=h  n=n  P0=P0
  Vessel (L-non-inverted derivative) : $bdroot/Vessel (L-non-inverted derivative)  VariantControl=choice == 7  l=l  r=r  h=h  n=n  P0=P0
  "Vessel (L-non-inverted) " : $bdroot/Vessel (L-non-inverted)   VariantControl=choice == 1  l=l  r=r  h=h  n=n  P0=P0
  Vessel (L-non-inverted) Volume control : $bdroot/Vessel (L-non-inverted) Volume control  VariantControl=choice == 8  l=l  r=r  h=h  n=n  P0=P0
  "Q_Output " : Outport
  "P_Input " : Outport  Port=2
  "Q_Input " : Outport  Port=3
  "P_Output " : Outport  Port=4
  V(t) : Outport  Port=5
  R : Outport  Port=6

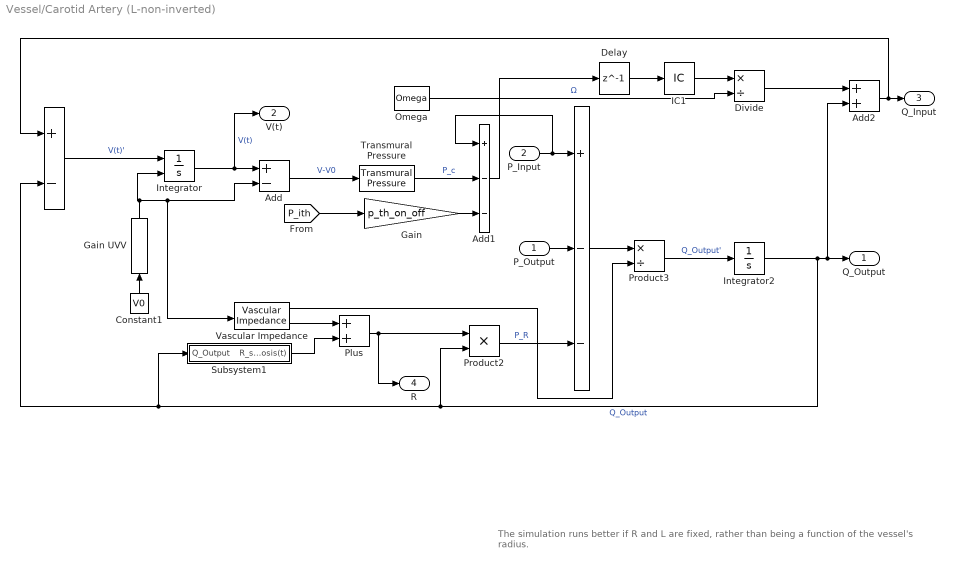
== system Vessel/Carotid Artery (L-non-inverted) ==
  note: The simulation runs better if R and L are fixed, rather than being a function of the vessel's radius.
  P_Output : Inport  Unit=mmHg
  P_Input : Inport  Port=2
  " " : Sum  Inputs=+--
  "   " : Sum  Inputs=+-
  Add : Sum  Inputs=+-
  Add1 : Sum  Inputs=+--
  Add2 : Sum
  Constant1 : Constant  Value=V0
  Delay : Delay  DelayLength=1  InitialCondition=P0
  Divide : Product  Inputs=*/
  Gain : Gain  Gain=p_th_on_off
  Gain UVV : $bdroot/Gain UVV  SystemSampleTime=-1  VariantActivationTime=update diagram  Latency=0  AutoFrameSizeCalculation=off
  IC1 : InitialCondition  Value=P0
  Integrator : Integrator  InitialConditionSource=external  LimitOutput=on  LowerSaturationLimit=0  ContinuousStateAttributes='Volume'
  Integrator2 : Integrator  LimitOutput=on  UpperSaturationLimit=4000  LowerSaturationLimit=-4000  ContinuousStateAttributes='Flow'
  Omega : $bdroot/Omega  SystemSampleTime=-1  VariantActivationTime=update diagram  Latency=0  AutoFrameSizeCalculation=off
  Plus : Sum
  Product2 : Product
  Product3 : Product  Inputs=*/
  Subsystem1 : Subsystem
  Transmural Pressure : $bdroot/Transmural Pressure  SystemSampleTime=-1  VariantActivationTime=update diagram  Latency=0  AutoFrameSizeCalculation=off
  Vascular Impedance : $bdroot/Vascular Impedance  SystemSampleTime=-1  VariantActivationTime=update diagram  Latency=0  AutoFrameSizeCalculation=off
  Q_Output : Outport
  V(t) : Outport  Port=2
  Q_Input : Outport  Port=3
  R : Outport  Port=4
  wires:
  Delay/1 -> IC1/1
  IC1/1 -> Divide/1
  Gain/1 -> Add1/3
  [P_ith] -> Gain/1
  Vascular Impedance/1 -> Product3/2
  Product3/1 -> Integrator2/1  "Q_Output'"
  "   "/1 -> Integrator/1  "V(t)'"
  Integrator/1 -> Add/1, V(t)/1  "V(t)"
  Add/1 -> Transmural Pressure/1  "V-V0"
  Product2/1 -> " "/3  "P_R"
  " "/1 -> Product3/1
  Add1/1 -> Delay/1
  Transmural Pressure/1 -> Add1/2  "P_c"
  Omega/1 -> Divide/2  "Ω"
  P_Output/1 -> " "/2
  Integrator2/1 -> Product2/2, Subsystem1/1(Q_Output), "   "/2, Add2/2, Q_Output/1  "Q_Output"
  Constant1/1 -> Gain UVV/1
  P_Input/1 -> " "/1, Add1/1
  Divide/1 -> Add2/1
  Gain UVV/1 -> Vascular Impedance/1, Add/2, Integrator/2
  Subsystem1/1(R_stenosis(t)) -> Plus/2
  Plus/1 -> Product2/1, R/1
  Vascular Impedance/2 -> Plus/1
  Add2/1 -> "   "/1, Q_Input/1

== system Vessel/Carotid Coarctation (L-inverted)1 ==
  note: The simulation runs better if R and L are fixed, rather than being a function of the vessel's radius.
  P_Output : Inport  Unit=mmHg
  P_Input : Inport  Port=2
  " " : Sum  Inputs=+--
  "   " : Sum  Inputs=+-
  Add : Sum  Inputs=+-
  Add1 : Sum  Inputs=+--
  Add2 : Sum
  Constant1 : Constant  Value=V0
  Delay : Delay  DelayLength=1  InitialCondition=P0
  Divide : Product  Inputs=*/
  Gain : Gain  Gain=0
  IC1 : InitialCondition  Value=P0
  Integrator : Integrator  InitialConditionSource=external  LimitOutput=on  LowerSaturationLimit=0  ContinuousStateAttributes='Volume'
  Integrator2 : Integrator  LimitOutput=on  UpperSaturationLimit=4000  LowerSaturationLimit=-4000  ContinuousStateAttributes='Flow'
  Omega : $bdroot/Omega  SystemSampleTime=-1  VariantActivationTime=update diagram  Latency=0  AutoFrameSizeCalculation=off
  Product2 : Product
  Product3 : Product  Inputs=*/
  Subsystem : $bdroot/Coarctation (L-non-inverted)/Subsystem  SystemSampleTime=-1  VariantActivationTime=update diagram  Latency=0  AutoFrameSizeCalculation=off
  Transmural Pressure : $bdroot/Transmural Pressure  SystemSampleTime=-1  VariantActivationTime=update diagram  Latency=0  AutoFrameSizeCalculation=off
  Vascular Impedance : $bdroot/Vascular Impedance  SystemSampleTime=-1  VariantActivationTime=update diagram  Latency=0  AutoFrameSizeCalculation=off
  Q_Output : Outport
  V(t) : Outport  Port=2
  Q_Input : Outport  Port=3
  R : Outport  Port=4
  wires:
  Divide/1 -> Q_Input/1, "   "/1
  P_Input/1 -> Add1/1, " "/1
  Constant1/1 -> Integrator/2, Vascular Impedance/1, Add/2
  Integrator2/1 -> Q_Output/1, Subsystem/1, "   "/2, Product2/2  "Q_Output"
  P_Output/1 -> " "/2
  Omega/1 -> Divide/2  "Ω"
  Transmural Pressure/1 -> Add1/2  "P_c"
  Add1/1 -> Delay/1
  " "/1 -> Product3/1
  Product2/1 -> " "/3  "P_R"
  Add/1 -> Transmural Pressure/1  "V-V0"
  Integrator/1 -> V(t)/1, Add/1  "V(t)"
  "   "/1 -> Integrator/1  "V(t)'"
  Product3/1 -> Integrator2/1  "Q_Output'"
  Vascular Impedance/2 -> Add2/1
  Vascular Impedance/1 -> Product3/2
  [P_ith] -> Gain/1
  Gain/1 -> Add1/3
  IC1/1 -> Divide/1
  Delay/1 -> IC1/1
  Subsystem/1 -> Add2/2
  Add2/1 -> R/1, Product2/1

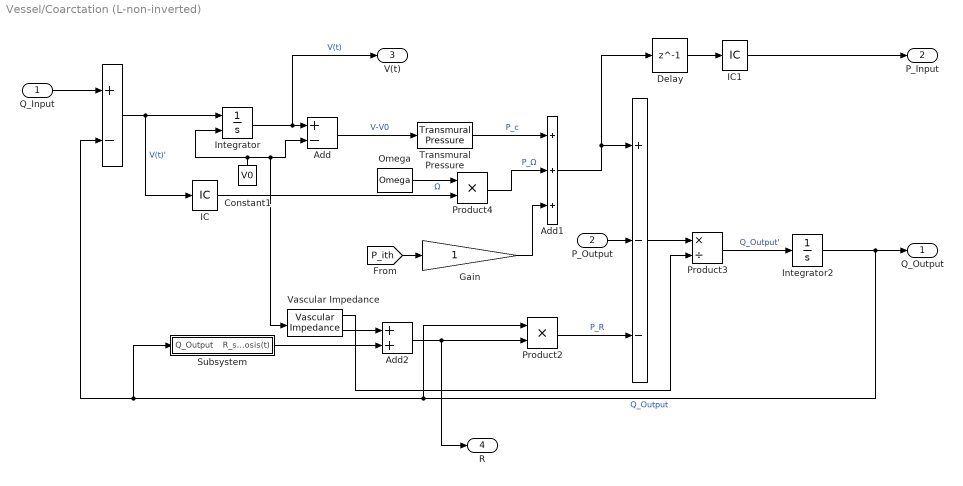
== system Vessel/Coarctation (L-non-inverted) ==
  Q_Input : Inport
  P_Output : Inport  Port=2  Unit=mmHg
  " " : Sum  Inputs=+--
  "   " : Sum  Inputs=+-
  Add : Sum  Inputs=+-
  Add1 : Sum  Inputs=+++
  Add2 : Sum
  Constant1 : Constant  Value=V0
  Delay : Delay  DelayLength=1  InitialCondition=P0
  Gain : Gain
  IC : InitialCondition  Value=0
  IC1 : InitialCondition  Value=P0
  Integrator : Integrator  InitialConditionSource=external  LimitOutput=on  LowerSaturationLimit=0  ContinuousStateAttributes='Volume'
  Integrator2 : Integrator  LimitOutput=on  UpperSaturationLimit=4000  LowerSaturationLimit=-4000  ContinuousStateAttributes='Flow'
  Omega : $bdroot/Omega  SystemSampleTime=-1  VariantActivationTime=update diagram  Latency=0  AutoFrameSizeCalculation=off
  Product2 : Product
  Product3 : Product  Inputs=*/
  Product4 : Product
  Subsystem : Subsystem
  Transmural Pressure : $bdroot/Transmural Pressure  SystemSampleTime=-1  VariantActivationTime=update diagram  Latency=0  AutoFrameSizeCalculation=off
  Vascular Impedance : $bdroot/Vascular Impedance  SystemSampleTime=-1  VariantActivationTime=update diagram  Latency=0  AutoFrameSizeCalculation=off
  Q_Output : Outport
  P_Input : Outport  Port=2
  V(t) : Outport  Port=3
  R : Outport  Port=4
  wires:
  Delay/1 -> IC1/1
  IC1/1 -> P_Input/1
  IC/1 -> Product4/2
  Gain/1 -> Add1/3
  [P_ith] -> Gain/1
  Vascular Impedance/1 -> Product3/2
  Vascular Impedance/2 -> Add2/1
  Product3/1 -> Integrator2/1  "Q_Output'"
  "   "/1 -> Integrator/1, IC/1  "V(t)'"
  Integrator/1 -> Add/1, V(t)/1  "V(t)"
  Add/1 -> Transmural Pressure/1  "V-V0"
  Product2/1 -> " "/3  "P_R"
  " "/1 -> Product3/1
  Add1/1 -> " "/1, Delay/1
  Transmural Pressure/1 -> Add1/1  "P_c"
  Q_Input/1 -> "   "/1
  Product4/1 -> Add1/2  "P_Ω"
  Omega/1 -> Product4/1  "Ω"
  P_Output/1 -> " "/2
  Integrator2/1 -> Subsystem/1(Q_Output), "   "/2, Product2/1, Q_Output/1  "Q_Output"
  Constant1/1 -> Vascular Impedance/1, Add/2, Integrator/2
  Add2/1 -> R/1, Product2/2
  Subsystem/1(R_stenosis(t)) -> Add2/2

== system Vessel/Coronary1 ==
  P_RA : Inport
  P_LV : Inport  Port=2
  P_aortic_root : Inport  Port=3
  Gain : Gain  Gain=1/R_ca
  Max : MinMax  Function=max  Inputs=2
  Subtract1 : Sum  Inputs=+-
  Q_Output : Outport
  wires:
  Gain/1 -> Q_Output/1
  Subtract1/1 -> Gain/1
  Max/1 -> Subtract1/2
  P_LV/1 -> Max/2
  P_aortic_root/1 -> Subtract1/1
  P_RA/1 -> Max/1

== system Vessel/Counter ==
  Add : Sum
  Constant : Constant  Value=Ts
  Unit Delay : UnitDelay  SampleTime=-1  HasFrameUpgradeWarning=on
  Unit Delay1 : UnitDelay  SampleTime=-1  HasFrameUpgradeWarning=on
  t : Outport
  wires:
  Unit Delay/1 -> Add/1
  Constant/1 -> Unit Delay/1
  Add/1 -> Unit Delay1/1
  Unit Delay1/1 -> Add/2, t/1
